simulink model "controller"  (R2019a)
settings: Solver=VariableStepAuto  StartTime=0.0  StopTime=10.0  RelTol=1e-3
values from neighbouring files (symbols this model uses):
  f_eff = 2.6*10^(-5)    (= 2.6e-05)    [PD.m]    (also in actuatorTest.m; inverseDyn-test.m)
  Jeff = double(Jeff_c(1))    [PD.m]
  k_T = 0.24    [PD.m]    (also in actuatorTest.m; inverseDyn-test.m)
  KD = double(K_D(1))    [PD.m]
  KI = double(K_I(1))    [PD.m]    (also in inverseDyn-test.m = 1)
  KP = double(K_P(1))    [PD.m]    (also in inverseDyn-test.m = 1)
  n = 53    [IndependentJoint.m]    (also in RNEA-test.m = length(q1); actuatorTest.m; newton.m = length(q1))
settings Model: Creator=sensei  LastModifiedBy=JanAriel

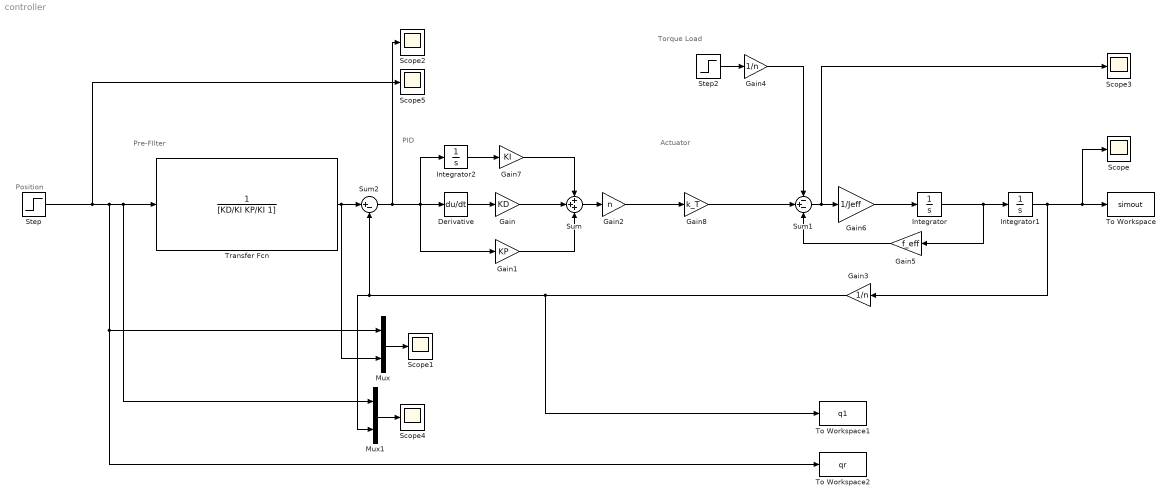
== system controller ==
  note: Position
  note: Actuator
  note: Pre-FIlter
  note: Torque Load
  note: PID
  Derivative : Derivative
  Gain : Gain  Gain=KD
  Gain1 : Gain  Gain=KP
  Gain2 : Gain  Gain=n
  Gain3 : Gain  Gain=1/n
  Gain4 : Gain  Gain=1/n
  Gain5 : Gain  Gain=f_eff
  Gain6 : Gain  Gain=1/Jeff
  Gain7 : Gain  Gain=KI
  Gain8 : Gain  Gain=k_T
  Integrator : Integrator
  Integrator1 : Integrator
  Integrator2 : Integrator
  Mux : Mux  Inputs=2
  Mux1 : Mux  Inputs=2
  Scope{,1..5} (6 alike) : Scope
  Step : Step  Time=0  After=0.35  SampleTime=0
  Step2 : Step  Time=5  After=6  SampleTime=0
  Sum : Sum  Inputs=+++
  Sum1 : Sum  Inputs=-+-
  Sum2 : Sum  Inputs=|+-
  To Workspace : ToWorkspace  VariableName=simout  SaveFormat=Structure With Time  SampleTime=-1
  To Workspace1 : ToWorkspace  VariableName=q1  SaveFormat=Structure With Time  SampleTime=-1
  To Workspace2 : ToWorkspace  VariableName=qr  SaveFormat=Structure With Time  SampleTime=-1
  Transfer Fcn : TransferFcn  Denominator=[KD/KI KP/KI 1]
  wires:
  Sum/1 -> Gain2/1
  Gain2/1 -> Gain8/1
  Integrator1/1 -> Scope/1, To Workspace/1, Gain3/1
  Integrator/1 -> Integrator1/1, Gain5/1
  Gain5/1 -> Sum1/3
  Step2/1 -> Gain4/1
  Gain4/1 -> Sum1/1
  Gain8/1 -> Sum1/2
  Gain6/1 -> Integrator/1
  Derivative/1 -> Gain/1
  Gain7/1 -> Sum/1
  Gain1/1 -> Sum/3
  Gain/1 -> Sum/2
  Integrator2/1 -> Gain7/1
  Sum2/1 -> Scope2/1, Integrator2/1, Derivative/1, Gain1/1
  Sum1/1 -> Scope3/1, Gain6/1
  Mux/1 -> Scope1/1
  Transfer Fcn/1 -> Sum2/1, Mux/2
  Gain3/1 -> To Workspace1/1, Sum2/2, Mux1/2
  Mux1/1 -> Scope4/1
  Step/1 -> Scope5/1, To Workspace2/1, Mux/1, Mux1/1, Transfer Fcn/1
